simulink model "PMSM_Wind_Turbine"  (R2021b)
settings: Solver=VariableStepAuto  StartTime=0  StopTime=2  RelTol=1e-3
undefined symbols (not defined in the file): Imag, Real
libraries: spsSeriesRLCLoadLib x4, spsVoltageMeasurementLib x4, spsCurrentMeasurementLib x3, spsGroundLib x1, spsPermanentMagnetSynchronousMachineLib x1, spsThreePhaseVIMeasurementLib x1, spsUniversalBridgeLib x1, spspowerguiLib x1
settings Model: Creator=TOP  LastModifiedBy=MahmoudAshraf
settings SolverCC: AlgebraicLoopSolver=TrustRegion
settings DataIOCC: ReturnWorkspaceOutputs=off
settings DebuggingCC: UnconnectedInputMsg=none  UnconnectedOutputMsg=none  UnconnectedLineMsg=none  SFMachineParentedDataDiag=warning  ArithmeticOperatorsInVariantConditions=warning
settings SFSimCC: SimUseLocalCustomCode=off  CustomCodeUndefinedFunction=UseInterfaceOnly
settings RTWCC: RTWUseLocalCustomCode=off

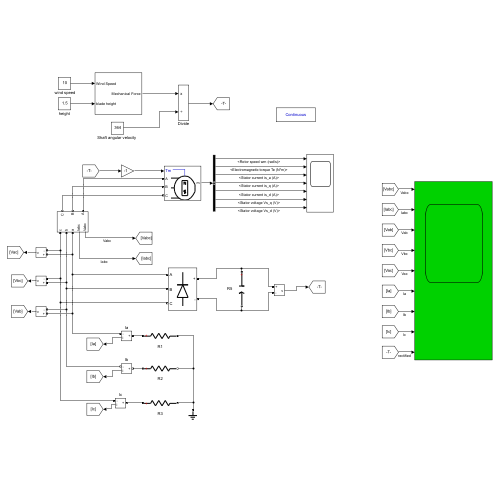
[thumbnail: Simulink's stored preview of the top-level diagram]
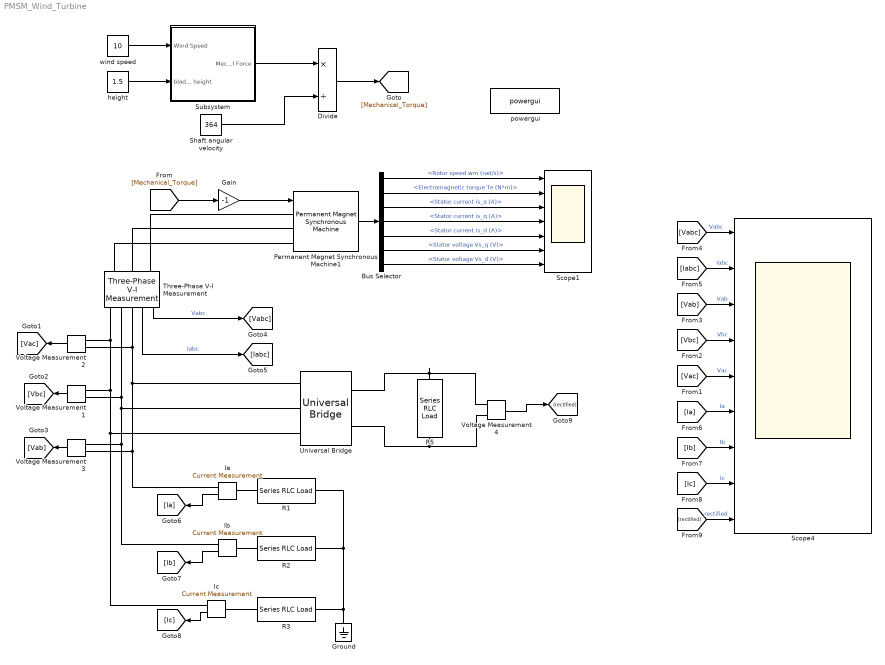
== system PMSM_Wind_Turbine ==
  " wind speed " : Constant  Value=10
  Bus Selector : BusSelector  OutputSignals=Rotor speed wm (rad/s),Electromagnetic torque Te (N*m),Stator current is_a (A),Stator current is_q (A),Stator current is_d (A),Stator voltage Vs_q (V),Stator voltage Vs_d (V)
  Divide : Product  Inputs=*/  OutMin=[1]  OutMax=[1000]
  Gain : Gain  Gain=-1
  Ground : spsGroundLib/Ground  LConnTagsString=a
  Ia : spsCurrentMeasurementLib/Current Measurement  PhasorSimulation=off  OutputType=Complex  PSBequivalent=0
  Ib : spsCurrentMeasurementLib/Current Measurement  PhasorSimulation=off  OutputType=Complex  PSBequivalent=0
  Ic : spsCurrentMeasurementLib/Current Measurement  PhasorSimulation=off  OutputType=Magnitude  PSBequivalent=0
  Permanent Magnet Synchronous Machine1 : spsPermanentMagnetSynchronousMachineLib/Permanent Magnet Synchronous Machine  NbPhases=3  FluxDistribution=Sinusoidal  RotorType=Round  MechanicalLoad=Torque Tm  PresetModel=No  ShowDetailedParameters=on  MeasurementBus=off  Resistance=0.18  Inductance=8.5e-3  dqInductances=[8.5e-3,8.5e-3]  La=0.000835  MachineConstant=Flux linkage established by magnets (V.s)  Flux=0.0714394  VoltageCst=51.8307  TorqueCst=0.42864  Flat=120  Mechanical=[0.000621417 0.000303448 4]  PolePairs=2  InitialConditions=[0,0, 0,0]  InitialConditions5ph=[0 0 0 0 0 0]  RefAngle=90 degrees behind phase A axis (modified Park)  IterativeDiscreteModel=Trapezoidal non iterative  TsBlock=-1  TsPowergui=0
  R1 : spsSeriesRLCLoadLib/Series RLC Load  LConnTagsString=a  RConnTagsString=__new0  NominalVoltage=230  NominalFrequency=50  ActivePower=10000  InductivePower=0  CapacitivePower=0  Setx0=off  InitialVoltage=0  SetiL0=off  InitialCurrent=0  Measurements=None  LoadType=constant Z
  R2 : spsSeriesRLCLoadLib/Series RLC Load  LConnTagsString=a  RConnTagsString=__new0  NominalVoltage=230  NominalFrequency=50  ActivePower=10000  InductivePower=0  CapacitivePower=0  Setx0=off  InitialVoltage=0  SetiL0=off  InitialCurrent=0  Measurements=None  LoadType=constant Z
  R3 : spsSeriesRLCLoadLib/Series RLC Load  LConnTagsString=a  RConnTagsString=__new0  NominalVoltage=230  NominalFrequency=50  ActivePower=10000  InductivePower=0  CapacitivePower=0  Setx0=off  InitialVoltage=0  SetiL0=off  InitialCurrent=0  Measurements=Branch voltage and current  LoadType=constant Z
  R5 : spsSeriesRLCLoadLib/Series RLC Load  LConnTagsString=a  RConnTagsString=__new0  NominalVoltage=230  NominalFrequency=50  ActivePower=0  InductivePower=0  CapacitivePower=100  Setx0=off  InitialVoltage=0  SetiL0=off  InitialCurrent=0  Measurements=Branch voltage and current  LoadType=constant Z
  Scope1 : Scope  NumInputPorts=7
  Scope4 : Scope  NumInputPorts=9
  "Shaft angular velocity " : Constant  Value=364
  Subsystem : Subsystem
  Three-Phase V-I Measurement : spsThreePhaseVIMeasurementLib/Three-Phase V-I Measurement  VoltageMeasurement=phase-to-phase  SetLabelV=off  LabelV=Vabc  Vpu=off  VpuLL=off  CurrentMeasurement=yes  SetLabelI=off  LabelI=Iabc  Ipu=off  Pbase=100e6  Vbase=500e3  OutputType=Complex  PhasorSimulation=off  PSBequivalent=0
  Universal Bridge : spsUniversalBridgeLib/Universal Bridge  Arms=3  SnubberResistance=1e5  SnubberCapacitance=inf  Device=Diodes  Ron=1e-3  Lon=0  ForwardVoltages="[  0  0  ]"  ForwardVoltage=0  GTOparameters=[ 10e-6 , 20e-6 ]  IGBTparameters=[ 1e-6 , 2e-6 ]  Measurements=None  Measurements_2=None  converterType=Rectifier
  Voltage Measurement1 : spsVoltageMeasurementLib/Voltage Measurement  PhasorSimulation=off  OutputType=Complex  PSBequivalent=0
  Voltage Measurement2 : spsVoltageMeasurementLib/Voltage Measurement  PhasorSimulation=off  OutputType=Complex  PSBequivalent=0
  Voltage Measurement3 : spsVoltageMeasurementLib/Voltage Measurement  PhasorSimulation=off  OutputType=Complex  PSBequivalent=0
  Voltage Measurement4 : spsVoltageMeasurementLib/Voltage Measurement  PhasorSimulation=off  OutputType=Real-Imag  PSBequivalent=0
  "height " : Constant  Value=1.5
  powergui : spspowerguiLib/powergui  Priority=1  SimulationMode=Continuous  SampleTime=50e-6  frequency=60  Iterations=50  frequencyindice=0  Pbase=100e6  ErrMax=1e-4  UnitsV=kV  UnitsW=MW  buscounter=0  FunctionMessages=off  echomessages=off  EnableUseOfTLC=off  CurrentSourceSwitches=off  DisableSnubberDevices=off  DisableRonSwitches=off  DisableVfSwitches=off  DisplayEquations=off  AutomaticDiscreteSolvers=off  SolverType=Tustin/Backward Euler (TBE)  Interpol=off  ExternalGateDelay=off  methode=off  Ts=100  x0status=blocks  SPID=on  SwTol=0  HookPort=off  NonlinearTolerance=1e-4  nMaxIteration=100  ContinueOnMaxIteration=off  RestoreLinks=warning  ResistiveCurrentMeasurement=off  Frange=[0:2:500]  Ylog=off  Xlog=on  ShowGrid=off  save=off  variable=ZData  structure=0  ZoomFFT=off  StartTime=0.0  cycles=1  DisplayStyle=1  fundamental=60  FreqAxis=off  MaxFrequency=1000  frequencyindicesteady=1  RmsSteady=2  display=off
  wires:
  "Shaft angular velocity "/1 -> Divide/2
  Gain/1 -> Permanent Magnet Synchronous Machine1/1
  Three-Phase V-I Measurement/2 -> [Iabc]  "Iabc"
  Three-Phase V-I Measurement/1 -> [Vabc]  "Vabc"
  Voltage Measurement4/1 -> [rectified]
  Permanent Magnet Synchronous Machine1/1 -> Bus Selector/1
  Bus Selector/1 -> Scope1/1  "<Rotor speed wm (rad/s)>"
  Bus Selector/2 -> Scope1/2  "<Electromagnetic torque Te (N*m)>"
  Bus Selector/3 -> Scope1/3  "<Stator current is_a (A)>"
  Bus Selector/4 -> Scope1/4  "<Stator current is_q (A)>"
  Bus Selector/5 -> Scope1/5  "<Stator current is_d (A)>"
  Bus Selector/6 -> Scope1/6  "<Stator voltage Vs_q (V)>"
  Bus Selector/7 -> Scope1/7  "<Stator voltage Vs_d (V)>"
  " wind speed "/1 -> Subsystem/1(Wind Speed)
  "height "/1 -> Subsystem/2(blade height)
  Subsystem/1(Mechanical Force) -> Divide/1
  Divide/1 -> [Mechanical_Torque]
  [Mechanical_Torque] -> Gain/1
  Voltage Measurement2/1 -> [Vac]
  Voltage Measurement1/1 -> [Vbc]
  Voltage Measurement3/1 -> [Vab]
  Ia/1 -> [Ia]
  Ib/1 -> [Ib]
  Ic/1 -> [Ic]
  [Vabc] -> Scope4/1  "Vabc"
  [Iabc] -> Scope4/2  "Iabc"
  [Vab] -> Scope4/3  "Vab"
  [Vbc] -> Scope4/4  "Vbc"
  [Vac] -> Scope4/5  "Vac"
  [Ia] -> Scope4/6  "Ia"
  [Ib] -> Scope4/7  "Ib"
  [Ic] -> Scope4/8  "Ic"
  [rectified] -> Scope4/9  "rectified"
  connections:
  Permanent Magnet Synchronous Machine1/LConn1 -- Three-Phase V-I Measurement/LConn1
  Permanent Magnet Synchronous Machine1/LConn3 -- Three-Phase V-I Measurement/LConn3
  R1/LConn1 -- Ia/LConn1
  R2/LConn1 -- Ib/LConn1
  Ic/LConn1 -- R3/LConn1
  R3/RConn1 -- R2/RConn1 -- R1/RConn1 -- Ground/LConn1
  Three-Phase V-I Measurement/RConn1 -- Voltage Measurement3/LConn1 -- Ia/RConn1 -- Universal Bridge/LConn1 -- Voltage Measurement2/LConn1
  Three-Phase V-I Measurement/RConn2 -- Voltage Measurement3/LConn2 -- Ib/RConn1 -- Universal Bridge/LConn2 -- Voltage Measurement1/LConn1
  Three-Phase V-I Measurement/RConn3 -- Voltage Measurement2/LConn2 -- Voltage Measurement1/LConn2 -- Ic/RConn1 -- Universal Bridge/LConn3
  Voltage Measurement4/LConn1 -- Universal Bridge/RConn1 -- R5/LConn1
  Universal Bridge/RConn2 -- R5/RConn1 -- Voltage Measurement4/LConn2
  Permanent Magnet Synchronous Machine1/LConn2 -- Three-Phase V-I Measurement/LConn2

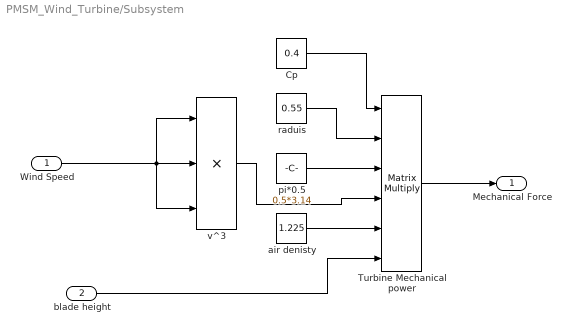
== system PMSM_Wind_Turbine/Subsystem ==
  Wind Speed : Inport
  blade height : Inport  Port=2
  " Turbine Mechanical power " : Product  Inputs=6  Multiplication=Matrix(*)
  Cp : Constant  Value=0.4
  air denisty : Constant  Value=1.225
  pi*0.5 : Constant  Value=0.5*3.14
  raduis : Constant  Value=0.55
  "v^3 " : Product  Inputs=***
  Mechanical Force : Outport
  wires:
  raduis/1 -> " Turbine Mechanical power "/2
  "v^3 "/1 -> " Turbine Mechanical power "/4
  " Turbine Mechanical power "/1 -> Mechanical Force/1
  Wind Speed/1 -> "v^3 "/3, "v^3 "/1, "v^3 "/2
  Cp/1 -> " Turbine Mechanical power "/1
  pi*0.5/1 -> " Turbine Mechanical power "/3
  blade height/1 -> " Turbine Mechanical power "/6
  air denisty/1 -> " Turbine Mechanical power "/5
